simulink model "lecture08_simulation"  (R2021a)
settings: Solver=VariableStepAuto  StartTime=0.0  StopTime=10.0  RelTol=1e-3
values from neighbouring files (symbols this model uses):
  Kp = piddata(Kps)    [lecture08_discrete_controllers.m]
  T = 0.1    [lecture08_discrete_controllers.m]
  Ti = 4    [lecture08_discrete_controllers.m]
  Tt = 0.1    [lecture08_discrete_controllers.m]
settings Model: Creator=Thomas Therkelsen  LastModifiedBy=Thomas Therkelsen

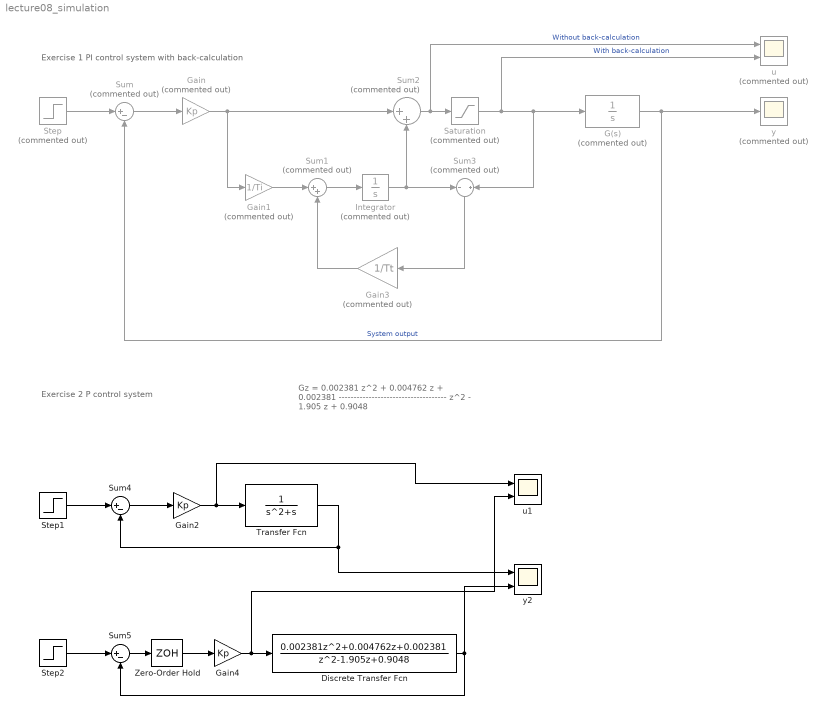
== system lecture08_simulation ==
  note: Gz =
      |
      |   0.002381 z^2 + 0.004762 z + 0.002381
      |   ------------------------------------
      |          z^2 - 1.905 z + 0.9048
  note: Exercise 1
      | PI control system with back-calculation
  note: Exercise 2
      | P control system
  Discrete Transfer Fcn : DiscreteTransferFcn  Numerator=[0.002381 0.004762 0.002381]  Denominator=[1 -1.905 0.9048]
  G(s) : TransferFcn  Commented=on  Denominator=[1 0]
  Gain : Gain  Commented=on  Gain=Kp
  Gain1 : Gain  Commented=on  Gain=1/Ti
  Gain2 : Gain  Gain=Kp
  Gain3 : Gain  Commented=on  Gain=1/Tt
  Gain4 : Gain  Gain=Kp
  Integrator : Integrator  Commented=on
  Saturation : Saturate  Commented=on  UpperLimit=1  LowerLimit=-1
  Step : Step  Commented=on  SampleTime=0
  Step1 : Step  SampleTime=0
  Step2 : Step  SampleTime=0
  Sum : Sum  Commented=on  Inputs=|+-
  Sum1 : Sum  Commented=on  Inputs=|++
  Sum2 : Sum  Commented=on  Inputs=|++
  Sum3 : Sum  Commented=on  Inputs=-||+
  Sum4 : Sum  Inputs=|+-
  Sum5 : Sum  Inputs=|+-
  Transfer Fcn : TransferFcn  Denominator=[1 1 0]
  Zero-Order Hold : ZeroOrderHold  SampleTime=T
  u : Scope  Commented=on  NumInputPorts=2
  u1 : Scope  NumInputPorts=2
  y : Scope  Commented=on
  y2 : Scope  NumInputPorts=2
  wires:
  Step/1 -> Sum/1
  Sum/1 -> Gain/1
  Gain/1 -> Sum2/1, Gain1/1
  Gain1/1 -> Sum1/1
  Sum1/1 -> Integrator/1
  Integrator/1 -> Sum3/1, Sum2/2
  Gain3/1 -> Sum1/2
  Sum2/1 -> u/1, Saturation/1  "Without back-calculation"
  Saturation/1 -> u/2, G(s)/1, Sum3/2  "With back-calculation"
  Sum3/1 -> Gain3/1
  G(s)/1 -> y/1, Sum/2  "System output"
  Gain2/1 -> u1/1, Transfer Fcn/1
  Step1/1 -> Sum4/1
  Sum4/1 -> Gain2/1
  Transfer Fcn/1 -> y2/1, Sum4/2
  Gain4/1 -> u1/2, Discrete Transfer Fcn/1
  Step2/1 -> Sum5/1
  Discrete Transfer Fcn/1 -> Sum5/2, y2/2
  Sum5/1 -> Zero-Order Hold/1
  Zero-Order Hold/1 -> Gain4/1
